simulink model "Robot_contour_array"  (R2021a)
settings: Solver=VariableStepAuto  StartTime=0.0  StopTime=1  RelTol=1e-3
values from neighbouring files (symbols this model uses):
  alfa1 = out.alfa1    [TotalPlot.m]
  alfa2 = out.alfa2    [TotalPlot.m]
  alfa3 = out.alfa3    [TotalPlot.m]
  X1 = out.X1    [TotalPlot.m]
  X2 = out.X2    [TotalPlot.m]
  X3 = out.X3    [TotalPlot.m]
  Y1 = out.Y1    [TotalPlot.m]
  Y2 = out.Y2    [TotalPlot.m]
  Y3 = out.Y3    [TotalPlot.m]

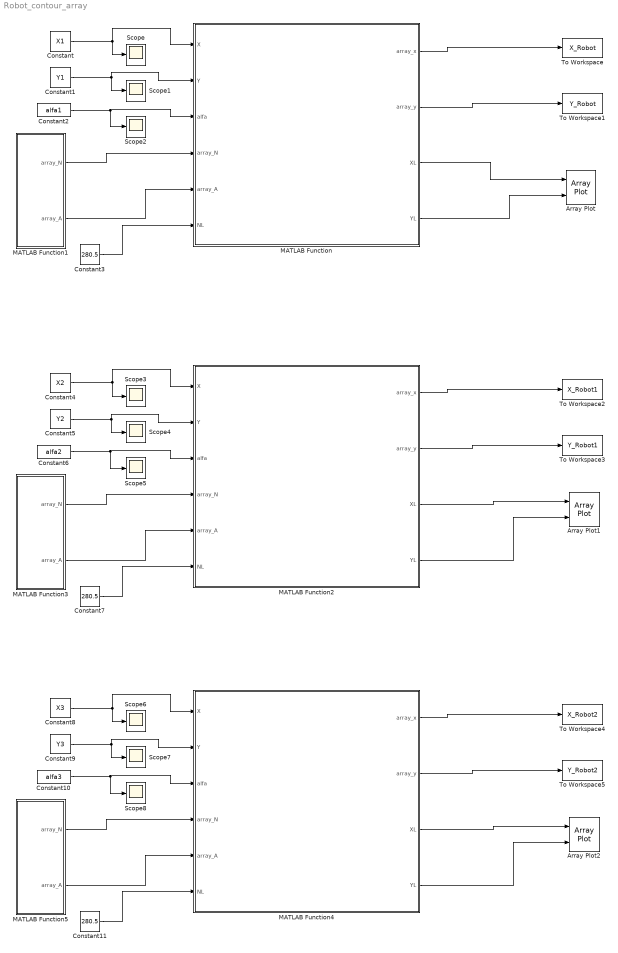
== system Robot_contour_array ==
  Array Plot : ArrayPlot  NumInputPorts=2  WindowPosition=[1.000000,49.000000,1536.000000,793.000000,]  YLimits=[1923.5505206074731,2473.1363836381797]  ShowLegend=on  DefaultConfigurationName=dsp.scopes.ArrayPlotBlockSpecification
  Array Plot1 : ArrayPlot  NumInputPorts=2  WindowPosition=[1.000000,49.000000,1536.000000,793.000000,]  YLimits=[5653.261151340503,7268.478623152074]  ShowLegend=on  DefaultConfigurationName=dsp.scopes.ArrayPlotBlockSpecification
  Array Plot2 : ArrayPlot  NumInputPorts=2  WindowPosition=[1.000000,49.000000,1536.000000,793.000000,]  YLimits=[5653.261151340503,7268.478623152074]  ShowLegend=on  DefaultConfigurationName=dsp.scopes.ArrayPlotBlockSpecification
  Constant : Constant  Value=X1  OutDataTypeStr=double  LockScale=on
  Constant1 : Constant  Value=Y1  OutDataTypeStr=double  LockScale=on
  Constant10 : Constant  Value=alfa3  OutDataTypeStr=double  LockScale=on
  Constant11 : Constant  Value=280.5
  Constant2 : Constant  Value=alfa1  OutDataTypeStr=double  LockScale=on
  Constant3 : Constant  Value=280.5
  Constant4 : Constant  Value=X2  OutDataTypeStr=double  LockScale=on
  Constant5 : Constant  Value=Y2  OutDataTypeStr=double  LockScale=on
  Constant6 : Constant  Value=alfa2  OutDataTypeStr=double  LockScale=on
  Constant7 : Constant  Value=280.5
  Constant8 : Constant  Value=X3  OutDataTypeStr=double  LockScale=on
  Constant9 : Constant  Value=Y3  OutDataTypeStr=double  LockScale=on
  MATLAB Function : MATLAB Function  TreatAsAtomicUnit=on
  MATLAB Function1 : MATLAB Function  TreatAsAtomicUnit=on
  MATLAB Function2 : MATLAB Function  TreatAsAtomicUnit=on
  MATLAB Function3 : MATLAB Function  TreatAsAtomicUnit=on
  MATLAB Function4 : MATLAB Function  TreatAsAtomicUnit=on
  MATLAB Function5 : MATLAB Function  TreatAsAtomicUnit=on
  Scope{,1..8} (9 alike) : Scope
  To Workspace : ToWorkspace  VariableName=X_Robot  SampleTime=1
  To Workspace1 : ToWorkspace  VariableName=Y_Robot  SampleTime=1
  To Workspace2 : ToWorkspace  VariableName=X_Robot1  SampleTime=1
  To Workspace3 : ToWorkspace  VariableName=Y_Robot1  SampleTime=1
  To Workspace4 : ToWorkspace  VariableName=X_Robot2  SampleTime=1
  To Workspace5 : ToWorkspace  VariableName=Y_Robot2  SampleTime=1
  wires:
  MATLAB Function1/1(array_N) -> MATLAB Function/4(array_N)
  MATLAB Function/1(array_x) -> To Workspace/1
  MATLAB Function/2(array_y) -> To Workspace1/1
  MATLAB Function1/2(array_A) -> MATLAB Function/5(array_A)
  Constant3/1 -> MATLAB Function/6(NL)
  MATLAB Function/3(XL) -> Array Plot/1
  Constant/1 -> Scope/1, MATLAB Function/1(X)
  Constant1/1 -> Scope1/1, MATLAB Function/2(Y)
  Constant2/1 -> Scope2/1, MATLAB Function/3(alfa)
  Constant5/1 -> Scope4/1, MATLAB Function2/2(Y)
  Constant4/1 -> Scope3/1, MATLAB Function2/1(X)
  MATLAB Function2/3(XL) -> Array Plot1/1
  MATLAB Function2/2(array_y) -> To Workspace3/1
  Constant6/1 -> Scope5/1, MATLAB Function2/3(alfa)
  MATLAB Function3/2(array_A) -> MATLAB Function2/5(array_A)
  Constant7/1 -> MATLAB Function2/6(NL)
  MATLAB Function3/1(array_N) -> MATLAB Function2/4(array_N)
  MATLAB Function2/1(array_x) -> To Workspace2/1
  MATLAB Function2/4(YL) -> Array Plot1/2
  MATLAB Function/4(YL) -> Array Plot/2
  Constant9/1 -> Scope7/1, MATLAB Function4/2(Y)
  MATLAB Function5/1(array_N) -> MATLAB Function4/4(array_N)
  MATLAB Function4/4(YL) -> Array Plot2/2
  MATLAB Function4/1(array_x) -> To Workspace4/1
  Constant11/1 -> MATLAB Function4/6(NL)
  MATLAB Function5/2(array_A) -> MATLAB Function4/5(array_A)
  MATLAB Function4/2(array_y) -> To Workspace5/1
  Constant10/1 -> Scope8/1, MATLAB Function4/3(alfa)
  MATLAB Function4/3(XL) -> Array Plot2/1
  Constant8/1 -> Scope6/1, MATLAB Function4/1(X)

== matlab function Robot_contour_array/MATLAB Function2 ==
function [array_x ,array_y,XL,YL ] = fcn(X,Y,alfa,array_N,array_A,NL)
a=size(X);
XL=zeros(a(1),1);
YL=zeros(a(1),1);
array_x=zeros(a(1),15);
array_y=zeros(a(1),15);
for n=1:a(1)

    for i=1:15 
    array_x(n,i)= X(n,1) + array_N(i)*cosd(alfa(n,1) -array_A(i));
    array_y(n,i)= Y(n,1) + array_N(i)*sind(alfa(n,1) -array_A(i));    

    end
XL(n,1)= X(n,1) + NL*cosd(alfa(n,1));
YL(n,1)= Y(n,1) + NL*sind(alfa(n,1));   
end

== matlab function Robot_contour_array/MATLAB Function3 ==
function [array_N,array_A]=fcn() 

array_N=[367.6,735.29,747.2,390.89,420.92,330.25,648.42,648.42,330.25,420.92,390.89,747.2,735.29,367.6,367.6];
array_A=[9.08,4.52,11.19,21.77,30.41,66.35,152.09,-152.09,-66.35,-30.41,-21.77,-11.19,-4.52,-9.08,9.08];

== matlab function Robot_contour_array/MATLAB Function4 ==
function [array_x ,array_y,XL,YL ] = fcn(X,Y,alfa,array_N,array_A,NL)
a=size(X);
XL=zeros(a(1),1);
YL=zeros(a(1),1);
array_x=zeros(a(1),15);
array_y=zeros(a(1),15);
for n=1:a(1)

    for i=1:15 
    array_x(n,i)= X(n,1) + array_N(i)*cosd(alfa(n,1) -array_A(i));
    array_y(n,i)= Y(n,1) + array_N(i)*sind(alfa(n,1) -array_A(i));    

    end
XL(n,1)= X(n,1) + NL*cosd(alfa(n,1));
YL(n,1)= Y(n,1) + NL*sind(alfa(n,1));   
end

== matlab function Robot_contour_array/MATLAB Function5 ==
function [array_N,array_A]=fcn() 

array_N=[367.6,735.29,747.2,390.89,420.92,330.25,648.42,648.42,330.25,420.92,390.89,747.2,735.29,367.6,367.6];
array_A=[9.08,4.52,11.19,21.77,30.41,66.35,152.09,-152.09,-66.35,-30.41,-21.77,-11.19,-4.52,-9.08,9.08];

== matlab function Robot_contour_array/MATLAB Function1 ==
function [array_N,array_A]=fcn() 

array_N=[367.6,735.29,747.2,390.89,420.92,330.25,648.42,648.42,330.25,420.92,390.89,747.2,735.29,367.6,367.6];
array_A=[9.08,4.52,11.19,21.77,30.41,66.35,152.09,-152.09,-66.35,-30.41,-21.77,-11.19,-4.52,-9.08,9.08];

== matlab function Robot_contour_array/MATLAB Function ==
function [array_x ,array_y,XL,YL ] = fcn(X,Y,alfa,array_N,array_A,NL)
a=size(X);
XL=zeros(a(1),1);
YL=zeros(a(1),1);
array_x=zeros(a(1),15);
array_y=zeros(a(1),15);
for n=1:a(1)

    for i=1:15 
    array_x(n,i)= X(n,1) + array_N(i)*cosd(alfa(n,1) -array_A(i));
    array_y(n,i)= Y(n,1) + array_N(i)*sind(alfa(n,1) -array_A(i));    

    end
XL(n,1)= X(n,1) + NL*cosd(alfa(n,1));
YL(n,1)= Y(n,1) + NL*sind(alfa(n,1));   
end
